simulink model "hyd_hyb_2_int_cont_Final_AMT"  (R2013b)
settings: Solver=ode4  StartTime=0  StopTime=3005  FixedStep=0.01  MaxStep=.4  RelTol=1e-8
InitFcn:
  | const_3_new
values from neighbouring files (symbols this model uses):
  Af = 6.3    [brk_enrg.m]    (also in brk_enrg_1.m)
  BSFC_906_205 = [3.5684 4.3466 5.1668 6.0769 6.988 7.8992 8.8104 9.7336 10.8548 11.9809 13.1112 14.2571 ... (663 elements, 39x17)]    [BSFC_map_906_205.mat]
  Cd = 0.55    [brk_enrg.m]    (also in brk_enrg_1.m)
  den = 1.202    [brk_enrg.m]    (also in brk_enrg_1.m)
  fr = 0.01    [brk_enrg.m]    (also in brk_enrg_1.m)
undefined symbols (not defined in the file or in its folder): clutchRise, down_spd_2, down_spd_3, down_spd_4, down_spd_c, Driving_Cycle, fuel_density, gearshift, I_wheel, Idle_spd_eng_906, M1_hydr, p_v_15, pmax_125, qv_125, Rw, sec_eng_sfc_map, T0, T1, T_max_906, T_min, TC_spd_ratio_max, teta_new_10, torque_convertor, Twait, up_spd_1, up_spd_2, up_spd_3, up_spd_c, v_p_10, v_p_15, v_p_5
libraries: neural x1742, fl_lib x43, nesl_utility x30, sdl_lib x14, simulink x4, simulink_need_slupdate x1
(part 3 of 26)

== system hyd_hyb_2_int_cont_Final_AMT/Transmission1/gear box/gear box/Clutch Control ==
  control : Inport
  1 : Constant
  2 : Constant  Value=2
  3 : Constant  Value=3
  4 : Constant  Value=4
  Add{,1..3} (4 alike) : Sum  Inputs=+-
  Enabled Subsystem1 : Subsystem  TreatAsAtomicUnit=on
  Enabled Subsystem2 : Subsystem  TreatAsAtomicUnit=on
  Enabled Subsystem3 : Subsystem  TreatAsAtomicUnit=on
  Enabled Subsystem4 : Subsystem  TreatAsAtomicUnit=on
  Mux2 : Mux
  disengahe : Constant  Value=-1
  engage : Constant
  selector{1..4} (4 alike) : Switch  Criteria=u2 ~= 0  Threshold=2300  ZeroCross=off
  Clutches : Outport
  wires:
  Mux2/1 -> Clutches/1
  engage/1 -> [engage]
  [disengage] -> selector1/1
  disengahe/1 -> [disengage]
  [engage] -> selector1/3
  control/1 -> Add/1, Add1/1, Add2/1, Add3/1
  Add/1 -> selector1/2
  1/1 -> Add/2
  [disengage] -> selector2/1
  [engage] -> selector2/3
  Add1/1 -> selector2/2
  2/1 -> Add1/2
  [disengage] -> selector3/1
  [engage] -> selector3/3
  Add2/1 -> selector3/2
  3/1 -> Add2/2
  [disengage] -> selector4/1
  [engage] -> selector4/3
  Add3/1 -> selector4/2
  4/1 -> Add3/2
  selector1/1 -> Enabled Subsystem1/Enable
  selector2/1 -> Enabled Subsystem2/Enable
  selector3/1 -> Enabled Subsystem3/Enable
  selector4/1 -> Enabled Subsystem4/Enable
  Enabled Subsystem1/1(clutch release) -> Mux2/1
  Enabled Subsystem2/1(clutch release) -> Mux2/2
  Enabled Subsystem3/1(clutch release) -> Mux2/3
  Enabled Subsystem4/1(clutch release) -> Mux2/4

== system hyd_hyb_2_int_cont_Final_AMT/controller1/online_fuz_clust/online_fuz_clus_main/new_feature_gen1 ==
  mem : Inport
  Clock : Clock
  MATLAB Function : MATLAB Function  TreatAsAtomicUnit=on
  Memory : Memory
  prc_spd_0_10 : Outport
  prc_spd_20_30 : Outport  Port=2
  max_acc : Outport  Port=3
  prc_acc_02_04 : Outport  Port=4
  prc_acc_06_08 : Outport  Port=5
  prc_dec_02_04 : Outport  Port=6
  prc_dec_06_08 : Outport  Port=7
  RPA : Outport  Port=8
  prc_spdacc_0_5 : Outport  Port=9
  PKE : Outport  Port=10
  wires:
  Clock/1 -> MATLAB Function/1(t)
  MATLAB Function/1(prc_spd_0_10) -> prc_spd_0_10/1
  MATLAB Function/2(prc_spd_20_30) -> prc_spd_20_30/1
  MATLAB Function/3(max_acc) -> max_acc/1
  MATLAB Function/4(prc_acc_02_04) -> prc_acc_02_04/1
  MATLAB Function/5(prc_acc_06_08) -> prc_acc_06_08/1
  MATLAB Function/6(prc_dec_02_04) -> prc_dec_02_04/1
  MATLAB Function/7(prc_dec_06_08) -> prc_dec_06_08/1
  MATLAB Function/8(rpa) -> RPA/1
  MATLAB Function/9(prc_av_0_5) -> prc_spdacc_0_5/1
  MATLAB Function/10(pke) -> PKE/1
  Memory/1 -> MATLAB Function/2(mem)
  mem/1 -> Memory/1

== system hyd_hyb_2_int_cont_Final_AMT/controller1/optimized controller/SOC under 0.5/col_c_d ==
  inps : Inport
  SOC : Inport  Port=2
  Switch : Switch  Criteria=u2 > Threshold  Threshold=0.4
  net_col_c_d_2_4 : Subsystem
  net_col_c_d_4_5 : Subsystem
  Out1 : Outport
  wires:
  inps/1 -> net_col_c_d_4_5/1(Input), net_col_c_d_2_4/1(Input)
  SOC/1 -> Switch/2
  net_col_c_d_4_5/1(Output) -> Switch/1
  net_col_c_d_2_4/1(Output) -> Switch/3
  Switch/1 -> Out1/1

== system hyd_hyb_2_int_cont_Final_AMT/controller1/optimized controller/SOC under 0.5/col_c_d1 ==
  inps : Inport
  SOC : Inport  Port=2
  Switch : Switch  Criteria=u2 > Threshold  Threshold=0.4
  net_col_c_d_2_4 : Subsystem
  net_col_c_d_4_5 : Subsystem
  Out1 : Outport
  wires:
  Switch/1 -> Out1/1
  net_col_c_d_2_4/1(Output) -> Switch/3
  net_col_c_d_4_5/1(Output) -> Switch/1
  SOC/1 -> Switch/2
  inps/1 -> net_col_c_d_2_4/1(Input), net_col_c_d_4_5/1(Input)

== system hyd_hyb_2_int_cont_Final_AMT/controller1/optimized controller/SOC under 0.5/col_e_f ==
  inps : Inport
  SOC : Inport  Port=2
  Switch : Switch  Criteria=u2 > Threshold  Threshold=0.4
  net_col_e_f_2_4 : Subsystem
  net_col_e_f_4_5 : Subsystem
  Out1 : Outport
  wires:
  inps/1 -> net_col_e_f_4_5/1(Input), net_col_e_f_2_4/1(Input)
  SOC/1 -> Switch/2
  net_col_e_f_4_5/1(Output) -> Switch/1
  net_col_e_f_2_4/1(Output) -> Switch/3
  Switch/1 -> Out1/1

== system hyd_hyb_2_int_cont_Final_AMT/controller1/optimized controller/SOC under 0.5/net_loc_rod_2_5 ==
  Input : Inport  PortDimensions=2
  Layer 1 : Subsystem
  Layer 2 : Subsystem
  Layer 3 : Subsystem
  Process Input 1 : Subsystem
  Process Output 1 : Subsystem
  Output : Outport  InitialOutput=0
  wires:
  Input/1 -> Process Input 1/1(x)
  Process Output 1/1(y) -> Output/1
  Process Input 1/1(p) -> Layer 1/1("p{1}")
  Layer 1/1("a{1}") -> [feedback1]
  [feedback1] -> Layer 2/1("a{1} ")
  Layer 2/1("a{2}") -> [feedback2]
  [feedback2] -> Layer 3/1("a{2} ")
  Layer 3/1("a{3}") -> Process Output 1/1(a)

== system hyd_hyb_2_int_cont_Final_AMT/controller1/optimized controller/SOC upper 0.5/SOC under 0.6 ==
  inps : Inport
  u_fuzz : Inport  Port=2
  Action Port : ActionPort  ActionType=then
  Demux : Demux
  Product{,1..3} (4 alike) : Product  RndMeth=Zero
  Saturation{1..4} (4 alike) : Saturate  UpperLimit=1  LowerLimit=0
  Sum : Sum  Inputs=++++
  net_col_a_b_5_6 : Subsystem
  net_col_c_d_5_6 : Subsystem
  net_col_e_f_5_6 : Subsystem
  net_loc_rod_5_6 : Subsystem
  T_ICE_opt : Outport
  wires:
  Sum/1 -> T_ICE_opt/1
  inps/1 -> net_col_c_d_5_6/1(Input), net_col_e_f_5_6/1(Input), net_loc_rod_5_6/1(Input), net_col_a_b_5_6/1(Input)
  net_loc_rod_5_6/1(Output) -> Saturation2/1
  Product/1 -> Sum/1
  net_col_c_d_5_6/1(Output) -> Saturation4/1
  net_col_a_b_5_6/1(Output) -> Saturation1/1
  net_col_e_f_5_6/1(Output) -> Saturation3/1
  Saturation2/1 -> Product/1
  Saturation1/1 -> Product1/1
  Saturation4/1 -> Product2/1
  Saturation3/1 -> Product3/1
  Demux/1 -> Product1/2
  Demux/2 -> Product2/2
  u_fuzz/1 -> Demux/1
  Demux/3 -> Product3/2
  Demux/4 -> Product/2
  Product3/1 -> Sum/4
  Product2/1 -> Sum/3
  Product1/1 -> Sum/2

== system hyd_hyb_2_int_cont_Final_AMT/controller1/optimized controller/SOC upper 0.5/SOC upper 0.6 ==
  In1 : Inport
  SOC : Inport  Port=2
  u_fuzz : Inport  Port=3
  Action Port : ActionPort  ActionType=else
  If : If  IfExpression=u1 <=0.7
  SOC under 0.7 : Subsystem  TreatAsAtomicUnit=on
  SOC upper 0.7 : Subsystem  TreatAsAtomicUnit=on
  Switch : Switch  Criteria=u2 > Threshold  Threshold=0.7
  T_ICE_opt : Outport
  wires:
  SOC/1 -> SOC upper 0.7/1(SOC), If/1, Switch/2
  In1/1 -> SOC under 0.7/1(inps), SOC upper 0.7/2(inps)
  If/1 -> SOC under 0.7/Action
  If/2 -> SOC upper 0.7/Action
  Switch/1 -> T_ICE_opt/1
  SOC upper 0.7/1(T_ICE_opt) -> Switch/1
  SOC under 0.7/1(T_ICE_opt) -> Switch/3
  u_fuzz/1 -> SOC under 0.7/2(u_fuzz), SOC upper 0.7/3(u_fuzz)

== system hyd_hyb_2_int_cont_Final_AMT/hydraulic transmission/PM_hydraulic_machine /eta estimator/eta_t ==
  qv : Inport
  delta_p : Inport  Port=2
  Pmax : Inport  Port=3
  Abs : Abs
  Abs1 : Abs
  Constant : Constant  Value=600
  Constant1 : Constant  Value=0
  Divide : Product  Inputs=*/
  Product : Product  RndMeth=Zero
  Product1 : Product  RndMeth=Zero
  Saturation : Saturate  UpperLimit=1  LowerLimit=0
  Saturation1 : Saturate  UpperLimit=inf  LowerLimit=0.0000001
  Scope : Scope
      settings: SaveName=ScopeData29
  Scope1 : Scope  NumInputPorts=2
      settings: TimeRange=2.2  YMin=-5~-5  YMax=5~5  SaveName=ScopeData30
  Scope2 : Scope
      settings: YMin=0  YMax=190  SaveName=ScopeData50
  Scope3 : Scope
      settings: YMin=0  YMax=190  SaveName=ScopeData51
  Switch : Switch  Threshold=1
  eta_t : Outport
  wires:
  qv/1 -> Product1/1, Abs1/1
  delta_p/1 -> Product1/2
  Pmax/1 -> Product/1
  Constant/1 -> Product/2
  Product1/1 -> Abs/1
  Abs/1 -> Divide/1, Scope1/1
  Product/1 -> Saturation1/1
  Abs1/1 -> Scope2/1, Switch/2
  Saturation/1 -> eta_t/1
  Switch/1 -> Saturation/1, Scope/1
  Divide/1 -> Switch/1, Scope3/1
  Constant1/1 -> Switch/3
  Saturation1/1 -> Divide/2, Scope1/2

== system hyd_hyb_2_int_cont_Final_AMT/hydraulic transmission/PM_hydraulic_machine /eta estimator/eta_v ==
  qv : Inport
  vg : Inport  Port=2
  n : Inport  Port=3
  Abs : Abs
  Abs1 : Abs
  Abs2 : Abs
  Constant : Constant  Value=1000
  Constant1 : Constant  Value=0.00001
  Divide : Product  Inputs=*/
  Product : Product  RndMeth=Zero
  Product1 : Product  RndMeth=Zero
  Saturation : Saturate  UpperLimit=1  LowerLimit=0.000001
  Saturation1 : Saturate  UpperLimit=inf  LowerLimit=0.0000001
  Scope : Scope  NumInputPorts=2
      settings: TimeRange=2  YMin=-5~-5  YMax=5~5  SaveName=ScopeData43
  Scope1 : Scope
      settings: TimeRange=2  SaveName=ScopeData44
  Scope2 : Scope  NumInputPorts=2
      settings: TimeRange=2  YMin=-5~-5  YMax=5~5  SaveName=ScopeData45
  Scope3 : Scope  NumInputPorts=2
      settings: TimeRange=2  YMin=-5~-5  YMax=5~5  SaveName=ScopeData46
  Scope4 : Scope
      settings: SaveName=ScopeData52
  Switch : Switch  Threshold=1
  eta_v : Outport
  wires:
  n/1 -> Product/1, Scope2/1
  vg/1 -> Product/2, Scope2/2
  qv/1 -> Scope3/1, Product1/1, Abs2/1
  Constant/1 -> Product1/2
  Product1/1 -> Abs/1
  Abs/1 -> Divide/1, Scope/1
  Product/1 -> Abs1/1
  Abs1/1 -> Scope/2, Saturation1/1
  Divide/1 -> Switch/1, Scope4/1
  Constant1/1 -> Switch/3
  Switch/1 -> Saturation/1, Scope1/1
  Saturation/1 -> eta_v/1
  Abs2/1 -> Switch/2
  Saturation1/1 -> Divide/2

== system hyd_hyb_2_int_cont_Final_AMT/hydraulic transmission/accumulator/max - min volume estimator/for 10 gal accumulator ==
  min_press(psi) : Inport
  max_press(psi) : Inport  Port=2
  pre_ch_press(psi) : Inport  Port=3
  Action Port : ActionPort  PropagateVarSize=During execution  ActionType=then
  Constant : Constant  Value=152
  Scope : Scope  NumInputPorts=2
      settings: YMin=-5~-5  YMax=5~5  SaveName=ScopeData40
  Scope1 : Scope  NumInputPorts=2
      settings: YMin=-5~-5  YMax=5~5  SaveName=ScopeData41
  in^3 to lit : Gain  Gain=16.387e-3
  in^3 to lit (1) : Gain  Gain=16.387e-3
  rexroth-1 : Lookup_n-D  BreakpointsForDimension1=[1000,1100,1200,1300,1400,1500,1600,1700,1800,1900,2000,2100,2200,2300,2400,2500,2600,2700,2800,2900,3000,3100,3200,3300,3400,3500,3600,3700,3800,3900,4000,4100,4200,4300,4400,4500,4600,4700,4800,4900,5000,5100,5200,5300,5400,5500,5600,5700,5800,5900,6000]  BreakpointsForDimension2=[1000,1400,2000]  Table=v_p_10  InputSameDT=on
  rexroth-10 : Lookup_n-D  BreakpointsForDimension1=[1000,1100,1200,1300,1400,1500,1600,1700,1800,1900,2000,2100,2200,2300,2400,2500,2600,2700,2800,2900,3000,3100,3200,3300,3400,3500,3600,3700,3800,3900,4000,4100,4200,4300,4400,4500,4600,4700,4800,4900,5000,5100,5200,5300,5400,5500,5600,5700,5800,5900,6000]  BreakpointsForDimension2=[1000,1400,2000]  Table=v_p_10  InputSameDT=on
  min_vol(lit) : Outport
  max_vol(lit) : Outport  Port=2
  accum_dry_mass ( kg ) : Outport  Port=3  InitialOutput=[0]
  wires:
  in^3 to lit/1 -> min_vol(lit)/1, Scope1/1
  rexroth-10/1 -> in^3 to lit (1)/1, Scope/2
  rexroth-1/1 -> in^3 to lit/1, Scope/1
  in^3 to lit (1)/1 -> max_vol(lit)/1, Scope1/2
  pre_ch_press(psi)/1 -> rexroth-10/2, rexroth-1/2
  min_press(psi)/1 -> rexroth-1/1
  max_press(psi)/1 -> rexroth-10/1
  Constant/1 -> accum_dry_mass ( kg )/1

== system hyd_hyb_2_int_cont_Final_AMT/hydraulic transmission/accumulator/max - min volume estimator/for 15 gal accumulator1 ==
  min_press(psi) : Inport
  max_press(psi) : Inport  Port=2
  pre_ch_press(psi) : Inport  Port=3
  Action Port : ActionPort  PropagateVarSize=During execution  ActionType=then
  Constant : Constant  Value=220
  Scope : Scope  NumInputPorts=2
      settings: YMin=-5~-5  YMax=5~5  SaveName=ScopeData38
  Scope1 : Scope  NumInputPorts=2
      settings: YMin=4.74484~24.0403  YMax=4.74484~24.0403  SaveName=ScopeData39
  in^3 to lit : Gain  Gain=16.387e-3
  in^3 to lit (1) : Gain  Gain=16.387e-3
  rexroth-1 : Lookup_n-D  BreakpointsForDimension1=[1000,1100,1200,1300,1400,1500,1600,1700,1800,1900,2000,2100,2200,2300,2400,2500,2600,2700,2800,2900,3000,3100,3200,3300,3400,3500,3600,3700,3800,3900,4000,4100,4200,4300,4400,4500,4600,4700,4800,4900,5000,5100,5200,5300,5400,5500,5600,5700,5800,5900,6000]  BreakpointsForDimension2=[1000,1400,2000]  Table=v_p_15  InputSameDT=on
  rexroth-15 : Lookup_n-D  BreakpointsForDimension1=[1000,1100,1200,1300,1400,1500,1600,1700,1800,1900,2000,2100,2200,2300,2400,2500,2600,2700,2800,2900,3000,3100,3200,3300,3400,3500,3600,3700,3800,3900,4000,4100,4200,4300,4400,4500,4600,4700,4800,4900,5000,5100,5200,5300,5400,5500,5600,5700,5800,5900,6000]  BreakpointsForDimension2=[1000,1400,2000]  Table=v_p_15  InputSameDT=on
  min_vol(lit) : Outport
  max_vol(lit) : Outport  Port=2
  accum_dry_mass ( kg ) : Outport  Port=3  InitialOutput=[0]
  wires:
  in^3 to lit/1 -> min_vol(lit)/1, Scope1/1
  rexroth-1/1 -> in^3 to lit (1)/1, Scope/2
  rexroth-15/1 -> in^3 to lit/1, Scope/1
  in^3 to lit (1)/1 -> max_vol(lit)/1, Scope1/2
  pre_ch_press(psi)/1 -> rexroth-15/2, rexroth-1/2
  min_press(psi)/1 -> rexroth-15/1
  max_press(psi)/1 -> rexroth-1/1
  Constant/1 -> accum_dry_mass ( kg )/1

== system hyd_hyb_2_int_cont_Final_AMT/hydraulic transmission/accumulator/max - min volume estimator/for 5 gal accumulator ==
  min_press(psi) : Inport
  max_press(psi) : Inport  Port=2
  pre_ch_press(psi) : Inport  Port=3
  Action Port : ActionPort  PropagateVarSize=During execution  ActionType=then
  Constant : Constant  Value=100
  Scope : Scope  NumInputPorts=2
      settings: YMin=-5~-5  YMax=5~5  SaveName=ScopeData27
  Scope1 : Scope  NumInputPorts=2
      settings: YMin=61.8714~626.852  YMax=61.8714~626.852  SaveName=ScopeData28
  in^3 to lit : Gain  Gain=16.387e-3
  in^3 to lit (1) : Gain  Gain=16.387e-3
  rexroth-1 : Lookup_n-D  BreakpointsForDimension1=[1000,1100,1200,1300,1400,1500,1600,1700,1800,1900,2000,2100,2200,2300,2400,2500,2600,2700,2800,2900,3000,3100,3200,3300,3400,3500,3600,3700,3800,3900,4000,4100,4200,4300,4400,4500,4600,4700,4800,4900,5000,5100,5200,5300,5400,5500,5600,5700,5800,5900,6000]  BreakpointsForDimension2=[1000,1400,2000]  Table=v_p_5  InputSameDT=on
  rexroth-5 : Lookup_n-D  BreakpointsForDimension1=[1000,1100,1200,1300,1400,1500,1600,1700,1800,1900,2000,2100,2200,2300,2400,2500,2600,2700,2800,2900,3000,3100,3200,3300,3400,3500,3600,3700,3800,3900,4000,4100,4200,4300,4400,4500,4600,4700,4800,4900,5000,5100,5200,5300,5400,5500,5600,5700,5800,5900,6000]  BreakpointsForDimension2=[1000,1400,2000]  Table=v_p_5  InputSameDT=on
  min_vol(lit) : Outport
  max_vol(lit) : Outport  Port=2
  accum_dry_mass ( kg ) : Outport  Port=3  InitialOutput=[0]
  wires:
  in^3 to lit/1 -> min_vol(lit)/1, Scope/1
  rexroth-1/1 -> in^3 to lit (1)/1, Scope1/2
  rexroth-5/1 -> in^3 to lit/1, Scope1/1
  in^3 to lit (1)/1 -> max_vol(lit)/1, Scope/2
  pre_ch_press(psi)/1 -> rexroth-5/2, rexroth-1/2
  min_press(psi)/1 -> rexroth-5/1
  max_press(psi)/1 -> rexroth-1/1
  Constant/1 -> accum_dry_mass ( kg )/1

== system hyd_hyb_2_int_cont_Final_AMT/Transmission1/Torque Convertor/main solver/Sensor(TC_in)/Motion sensor ==
  Ideal Rotational Motion Sensor : fl_lib/Mechanical/Mechanical Sensors/Ideal Rotational Motion Sensor  offset=0 rad  w_Log=off  t_Log=off  phi_Log=off  LocalVarNames=|w|t|phi  LocalVarDescs=|w|t|phi  LocalVarLogging=[]
  MRR : fl_lib/Mechanical/Rotational Elements/Mechanical Rotational Reference  t_Log=off  LocalVarNames=|t  LocalVarDescs=|t  LocalVarLogging=[]
  PS-Simulink Converter : nesl_utility/PS-Simulink Converter  PhysicalDomain=network_engine_domain  SubClassName=ps_output  LeftPortType=input  RightPortType=output  PseudoPeriodic=off  Frequencies=[]  Unit=rad/s  AffineConversion=off
  A : PMIOPort  Port=1  Side=Left
  W : Outport
  wires:
  PS-Simulink Converter/1 -> W/1
  connections:
  A/RConn1 -- Ideal Rotational Motion Sensor/LConn1
  Ideal Rotational Motion Sensor/RConn2 -- PS-Simulink Converter/LConn1
  MRR/LConn1 -- Ideal Rotational Motion Sensor/RConn1

== system hyd_hyb_2_int_cont_Final_AMT/Transmission1/Torque Convertor/main solver/Sensor(TC_in)/Torque sensor ==
  PS2S : nesl_utility/PS-Simulink Converter  PhysicalDomain=network_engine_domain  SubClassName=ps_output  LeftPortType=input  RightPortType=output  PseudoPeriodic=off  Frequencies=[]  Unit=1  AffineConversion=off
  Torque Sensor : fl_lib/Mechanical/Mechanical Sensors/Ideal Torque Sensor  w_Log=off  t_Log=off  LocalVarNames=|w|t  LocalVarDescs=|w|t  LocalVarLogging=[]
  B : PMIOPort  Port=1  Side=Right
  A : PMIOPort  Port=2  Side=Left
  T : Outport
  wires:
  PS2S/1 -> T/1
  connections:
  A/RConn1 -- Torque Sensor/LConn1
  B/RConn1 -- Torque Sensor/RConn1
  Torque Sensor/RConn2 -- PS2S/LConn1

== system hyd_hyb_2_int_cont_Final_AMT/Transmission1/Torque Convertor/main solver/Sensor(TC_out)/Motion sensor ==
  Ideal Rotational Motion Sensor : fl_lib/Mechanical/Mechanical Sensors/Ideal Rotational Motion Sensor  offset=0 rad  w_Log=off  t_Log=off  phi_Log=off  LocalVarNames=|w|t|phi  LocalVarDescs=|w|t|phi  LocalVarLogging=[]
  MRR : fl_lib/Mechanical/Rotational Elements/Mechanical Rotational Reference  t_Log=off  LocalVarNames=|t  LocalVarDescs=|t  LocalVarLogging=[]
  PS-Simulink Converter : nesl_utility/PS-Simulink Converter  PhysicalDomain=network_engine_domain  SubClassName=ps_output  LeftPortType=input  RightPortType=output  PseudoPeriodic=off  Frequencies=[]  Unit=rad/s  AffineConversion=off
  A : PMIOPort  Port=1  Side=Left
  W : Outport
  wires:
  PS-Simulink Converter/1 -> W/1
  connections:
  MRR/LConn1 -- Ideal Rotational Motion Sensor/RConn1
  Ideal Rotational Motion Sensor/RConn2 -- PS-Simulink Converter/LConn1
  A/RConn1 -- Ideal Rotational Motion Sensor/LConn1

== system hyd_hyb_2_int_cont_Final_AMT/Transmission1/Torque Convertor/main solver/Sensor(TC_out)/Torque sensor ==
  PS2S : nesl_utility/PS-Simulink Converter  PhysicalDomain=network_engine_domain  SubClassName=ps_output  LeftPortType=input  RightPortType=output  PseudoPeriodic=off  Frequencies=[]  Unit=1  AffineConversion=off
  Torque Sensor : fl_lib/Mechanical/Mechanical Sensors/Ideal Torque Sensor  w_Log=off  t_Log=off  LocalVarNames=|w|t  LocalVarDescs=|w|t  LocalVarLogging=[]
  B : PMIOPort  Port=1  Side=Right
  A : PMIOPort  Port=2  Side=Left
  T : Outport
  wires:
  PS2S/1 -> T/1
  connections:
  Torque Sensor/RConn2 -- PS2S/LConn1
  B/RConn1 -- Torque Sensor/RConn1
  A/RConn1 -- Torque Sensor/LConn1

== system hyd_hyb_2_int_cont_Final_AMT/Transmission1/gear box/gear box/Clutch Control/Enabled Subsystem1 ==
  Enable : EnablePort  StatesWhenEnabling=reset  PropagateVarSize=During execution
  Clutch A Actuator : TransferFcn  Numerator=[1/clutchRise]  Denominator=[1 1/clutchRise]
  engage : Constant
  clutch release : Outport  OutputWhenDisabled=reset  InitialOutput=[0]
  wires:
  engage/1 -> Clutch A Actuator/1
  Clutch A Actuator/1 -> clutch release/1

== system hyd_hyb_2_int_cont_Final_AMT/Transmission1/gear box/gear box/Clutch Control/Enabled Subsystem2 ==
  Enable : EnablePort  StatesWhenEnabling=reset  PropagateVarSize=During execution
  Clutch A Actuator : TransferFcn  Numerator=[1/clutchRise]  Denominator=[1 1/clutchRise]
  engage : Constant
  clutch release : Outport  OutputWhenDisabled=reset  InitialOutput=[0]
  wires:
  Clutch A Actuator/1 -> clutch release/1
  engage/1 -> Clutch A Actuator/1

== system hyd_hyb_2_int_cont_Final_AMT/Transmission1/gear box/gear box/Clutch Control/Enabled Subsystem3 ==
  Enable : EnablePort  StatesWhenEnabling=reset  PropagateVarSize=During execution
  Clutch A Actuator : TransferFcn  Numerator=[1/clutchRise]  Denominator=[1 1/clutchRise]
  engage : Constant
  clutch release : Outport  OutputWhenDisabled=reset  InitialOutput=[0]
  wires:
  engage/1 -> Clutch A Actuator/1
  Clutch A Actuator/1 -> clutch release/1

== system hyd_hyb_2_int_cont_Final_AMT/Transmission1/gear box/gear box/Clutch Control/Enabled Subsystem4 ==
  Enable : EnablePort  StatesWhenEnabling=reset  PropagateVarSize=During execution
  Clutch A Actuator : TransferFcn  Numerator=[1/clutchRise]  Denominator=[1 1/clutchRise]
  engage : Constant
  clutch release : Outport  OutputWhenDisabled=reset  InitialOutput=[0]
  wires:
  Clutch A Actuator/1 -> clutch release/1
  engage/1 -> Clutch A Actuator/1

== system hyd_hyb_2_int_cont_Final_AMT/controller1/optimized controller/SOC under 0.5/col_c_d/net_col_c_d_2_4 ==
  Input : Inport  PortDimensions=2
  Layer 1 : Subsystem
  Layer 2 : Subsystem
  Layer 3 : Subsystem
  Process Input 1 : Subsystem
  Process Output 1 : Subsystem
  Output : Outport  InitialOutput=0
  wires:
  Input/1 -> Process Input 1/1(x)
  Process Output 1/1(y) -> Output/1
  Process Input 1/1(p) -> Layer 1/1("p{1}")
  Layer 1/1("a{1}") -> [feedback1]
  [feedback1] -> Layer 2/1("a{1} ")
  Layer 2/1("a{2}") -> [feedback2]
  [feedback2] -> Layer 3/1("a{2} ")
  Layer 3/1("a{3}") -> Process Output 1/1(a)

== system hyd_hyb_2_int_cont_Final_AMT/controller1/optimized controller/SOC under 0.5/col_c_d/net_col_c_d_4_5 ==
  Input : Inport  PortDimensions=2
  Layer 1 : Subsystem
  Layer 2 : Subsystem
  Layer 3 : Subsystem
  Process Input 1 : Subsystem
  Process Output 1 : Subsystem
  Output : Outport  InitialOutput=0
  wires:
  Input/1 -> Process Input 1/1(x)
  Process Output 1/1(y) -> Output/1
  Process Input 1/1(p) -> Layer 1/1("p{1}")
  Layer 1/1("a{1}") -> [feedback1]
  [feedback1] -> Layer 2/1("a{1} ")
  Layer 2/1("a{2}") -> [feedback2]
  [feedback2] -> Layer 3/1("a{2} ")
  Layer 3/1("a{3}") -> Process Output 1/1(a)

== system hyd_hyb_2_int_cont_Final_AMT/controller1/optimized controller/SOC under 0.5/col_c_d1/net_col_c_d_2_4 ==
  Input : Inport  PortDimensions=2
  Layer 1 : Subsystem
  Layer 2 : Subsystem
  Layer 3 : Subsystem
  Process Input 1 : Subsystem
  Process Output 1 : Subsystem
  Output : Outport  InitialOutput=0
  wires:
  Layer 3/1("a{3}") -> Process Output 1/1(a)
  [feedback2] -> Layer 3/1("a{2} ")
  Layer 2/1("a{2}") -> [feedback2]
  [feedback1] -> Layer 2/1("a{1} ")
  Layer 1/1("a{1}") -> [feedback1]
  Process Input 1/1(p) -> Layer 1/1("p{1}")
  Process Output 1/1(y) -> Output/1
  Input/1 -> Process Input 1/1(x)

== system hyd_hyb_2_int_cont_Final_AMT/controller1/optimized controller/SOC under 0.5/col_c_d1/net_col_c_d_4_5 ==
  Input : Inport  PortDimensions=2
  Layer 1 : Subsystem
  Layer 2 : Subsystem
  Layer 3 : Subsystem
  Process Input 1 : Subsystem
  Process Output 1 : Subsystem
  Output : Outport  InitialOutput=0
  wires:
  Layer 3/1("a{3}") -> Process Output 1/1(a)
  [feedback2] -> Layer 3/1("a{2} ")
  Layer 2/1("a{2}") -> [feedback2]
  [feedback1] -> Layer 2/1("a{1} ")
  Layer 1/1("a{1}") -> [feedback1]
  Process Input 1/1(p) -> Layer 1/1("p{1}")
  Process Output 1/1(y) -> Output/1
  Input/1 -> Process Input 1/1(x)

== system hyd_hyb_2_int_cont_Final_AMT/controller1/optimized controller/SOC under 0.5/col_e_f/net_col_e_f_2_4 ==
  Input : Inport  PortDimensions=2
  Layer 1 : Subsystem
  Layer 2 : Subsystem
  Layer 3 : Subsystem
  Process Input 1 : Subsystem
  Process Output 1 : Subsystem
  Output : Outport  InitialOutput=0
  wires:
  Input/1 -> Process Input 1/1(x)
  Process Output 1/1(y) -> Output/1
  Process Input 1/1(p) -> Layer 1/1("p{1}")
  Layer 1/1("a{1}") -> [feedback1]
  [feedback1] -> Layer 2/1("a{1} ")
  Layer 2/1("a{2}") -> [feedback2]
  [feedback2] -> Layer 3/1("a{2} ")
  Layer 3/1("a{3}") -> Process Output 1/1(a)

== system hyd_hyb_2_int_cont_Final_AMT/controller1/optimized controller/SOC under 0.5/col_e_f/net_col_e_f_4_5 ==
  Input : Inport  PortDimensions=2
  Layer 1 : Subsystem
  Layer 2 : Subsystem
  Layer 3 : Subsystem
  Process Input 1 : Subsystem
  Process Output 1 : Subsystem
  Output : Outport  InitialOutput=0
  wires:
  Input/1 -> Process Input 1/1(x)
  Process Output 1/1(y) -> Output/1
  Process Input 1/1(p) -> Layer 1/1("p{1}")
  Layer 1/1("a{1}") -> [feedback1]
  [feedback1] -> Layer 2/1("a{1} ")
  Layer 2/1("a{2}") -> [feedback2]
  [feedback2] -> Layer 3/1("a{2} ")
  Layer 3/1("a{3}") -> Process Output 1/1(a)

== system hyd_hyb_2_int_cont_Final_AMT/controller1/optimized controller/SOC under 0.5/net_loc_rod_2_5/Layer 1 ==
  "p{1}" : Inport  PortDimensions=2
  Delays 1 : Subsystem
  "IW{1,1}" : Subsystem
  "b{1}" : Constant  Value=[-4.427231660818169;3.456636280494104;2.4300449872666854;1.4410928325775507;-0.49232939607411785;-0.49242330153496311;1.5258039114342512;-2.4759475246010565;3.4877744812530702;-4.4171792578500666]
  netsum : Sum  Inputs=2  SaturateOnIntegerOverflow=on  InputSameDT=on  OutDataTypeStr=Inherit: Same as first input
  tansig : neural/Transfer Functions/tansig
  "a{1}" : Outport  InitialOutput=[0;0;0;0;0;0;0;0;0;0]
  wires:
  "p{1}"/1 -> Delays 1/1("p{1}")
  Delays 1/1("pd{1,1}") -> "IW{1,1}"/1("pd{1,1}")
  "IW{1,1}"/1("iz{1,1}") -> netsum/1
  "b{1}"/1 -> netsum/2
  netsum/1 -> tansig/1
  tansig/1 -> "a{1}"/1

== system hyd_hyb_2_int_cont_Final_AMT/controller1/optimized controller/SOC under 0.5/net_loc_rod_2_5/Layer 2 ==
  "a{1} " : Inport  PortDimensions=10
  Delays 1 : Subsystem
  "LW{2,1}" : Subsystem
  "b{2}" : Constant  Value=[-1.8283395045760578;-1.5112791815228035;-1.3096453352155384;0.99927747204973882;-0.87070649425908642;0.57038205764658179;0.26248556891103664;0.037384065008415478;-0.25474765773298769;-0.5223912617711548;0.79462611488080304;0.93340606123125525;-1.2890933117577059;1.5735286477660981;-1.8440196925158161]
  netsum : Sum  Inputs=2  SaturateOnIntegerOverflow=on  InputSameDT=on  OutDataTypeStr=Inherit: Same as first input
  tansig : neural/Transfer Functions/tansig
  "a{2}" : Outport  InitialOutput=[0;0;0;0;0;0;0;0;0;0;0;0;0;0;0]
  wires:
  "a{1} "/1 -> Delays 1/1("p{2}")
  Delays 1/1("pd{2,1}") -> "LW{2,1}"/1("ad{2,1}")
  "LW{2,1}"/1("lz{2,1}") -> netsum/1
  "b{2}"/1 -> netsum/2
  netsum/1 -> tansig/1
  tansig/1 -> "a{2}"/1

== system hyd_hyb_2_int_cont_Final_AMT/controller1/optimized controller/SOC under 0.5/net_loc_rod_2_5/Layer 3 ==
  "a{2} " : Inport  PortDimensions=15
  Delays 1 : Subsystem
  "LW{3,2}" : Subsystem
  "b{3}" : Constant  Value=0.060410481787306604
  netsum : Sum  Inputs=2  SaturateOnIntegerOverflow=on  InputSameDT=on  OutDataTypeStr=Inherit: Same as first input
  purelin : neural/Transfer Functions/purelin
  "a{3}" : Outport  InitialOutput=0
  wires:
  "a{2} "/1 -> Delays 1/1("p{3}")
  Delays 1/1("pd{3,2}") -> "LW{3,2}"/1("ad{3,2}")
  "LW{3,2}"/1("lz{3,2}") -> netsum/1
  "b{3}"/1 -> netsum/2
  netsum/1 -> purelin/1
  purelin/1 -> "a{3}"/1

== system hyd_hyb_2_int_cont_Final_AMT/controller1/optimized controller/SOC under 0.5/net_loc_rod_2_5/Process Input 1 ==
  x : Inport  PortDimensions=2
  fixunknowns : neural/Processing Functions/fixunknowns  inputSize=2  indices=[1 2]
  mapminmax : neural/Processing Functions/mapminmax  xmin=[0.0022593599778436804;0.375]  xmax=[1;0.48752699999999999]  ymin=-1  ymax=1
  removeconstantrows : neural/Processing Functions/removeconstantrows  inputSize=2  keep=[1 2]
  p : Outport  PortDimensions=2
  wires:
  x/1 -> fixunknowns/1
  fixunknowns/1 -> removeconstantrows/1
  removeconstantrows/1 -> mapminmax/1
  mapminmax/1 -> p/1

== system hyd_hyb_2_int_cont_Final_AMT/controller1/optimized controller/SOC under 0.5/net_loc_rod_2_5/Process Output 1 ==
  a : Inport  PortDimensions=1
  mapminmax_reverse : neural/Processing Functions/mapminmax_reverse  xmin=0  xmax=0.71867283838575113  ymin=-1  ymax=1
  removeconstantrows_reverse : neural/Processing Functions/removeconstantrows_reverse  inputSize=1  constants=zeros(0,1)  rearrange=1
  y : Outport  PortDimensions=1
  wires:
  a/1 -> mapminmax_reverse/1
  mapminmax_reverse/1 -> removeconstantrows_reverse/1
  removeconstantrows_reverse/1 -> y/1

== system hyd_hyb_2_int_cont_Final_AMT/controller1/optimized controller/SOC upper 0.5/SOC under 0.6/net_col_a_b_5_6 ==
  Input : Inport  PortDimensions=2
  Layer 1 : Subsystem
  Layer 2 : Subsystem
  Layer 3 : Subsystem
  Process Input 1 : Subsystem
  Process Output 1 : Subsystem
  Output : Outport  InitialOutput=0
  wires:
  Input/1 -> Process Input 1/1(x)
  Process Output 1/1(y) -> Output/1
  Process Input 1/1(p) -> Layer 1/1("p{1}")
  Layer 1/1("a{1}") -> [feedback1]
  [feedback1] -> Layer 2/1("a{1} ")
  Layer 2/1("a{2}") -> [feedback2]
  [feedback2] -> Layer 3/1("a{2} ")
  Layer 3/1("a{3}") -> Process Output 1/1(a)

== system hyd_hyb_2_int_cont_Final_AMT/controller1/optimized controller/SOC upper 0.5/SOC under 0.6/net_col_c_d_5_6 ==
  Input : Inport  PortDimensions=2
  Layer 1 : Subsystem
  Layer 2 : Subsystem
  Layer 3 : Subsystem
  Process Input 1 : Subsystem
  Process Output 1 : Subsystem
  Output : Outport  InitialOutput=0
  wires:
  Input/1 -> Process Input 1/1(x)
  Process Output 1/1(y) -> Output/1
  Process Input 1/1(p) -> Layer 1/1("p{1}")
  Layer 1/1("a{1}") -> [feedback1]
  [feedback1] -> Layer 2/1("a{1} ")
  Layer 2/1("a{2}") -> [feedback2]
  [feedback2] -> Layer 3/1("a{2} ")
  Layer 3/1("a{3}") -> Process Output 1/1(a)

== system hyd_hyb_2_int_cont_Final_AMT/controller1/optimized controller/SOC upper 0.5/SOC under 0.6/net_col_e_f_5_6 ==
  Input : Inport  PortDimensions=2
  Layer 1 : Subsystem
  Layer 2 : Subsystem
  Layer 3 : Subsystem
  Process Input 1 : Subsystem
  Process Output 1 : Subsystem
  Output : Outport  InitialOutput=0
  wires:
  Input/1 -> Process Input 1/1(x)
  Process Output 1/1(y) -> Output/1
  Process Input 1/1(p) -> Layer 1/1("p{1}")
  Layer 1/1("a{1}") -> [feedback1]
  [feedback1] -> Layer 2/1("a{1} ")
  Layer 2/1("a{2}") -> [feedback2]
  [feedback2] -> Layer 3/1("a{2} ")
  Layer 3/1("a{3}") -> Process Output 1/1(a)

== system hyd_hyb_2_int_cont_Final_AMT/controller1/optimized controller/SOC upper 0.5/SOC under 0.6/net_loc_rod_5_6 ==
  Input : Inport  PortDimensions=2
  Layer 1 : Subsystem
  Layer 2 : Subsystem
  Layer 3 : Subsystem
  Process Input 1 : Subsystem
  Process Output 1 : Subsystem
  Output : Outport  InitialOutput=0
  wires:
  Input/1 -> Process Input 1/1(x)
  Process Output 1/1(y) -> Output/1
  Process Input 1/1(p) -> Layer 1/1("p{1}")
  Layer 1/1("a{1}") -> [feedback1]
  [feedback1] -> Layer 2/1("a{1} ")
  Layer 2/1("a{2}") -> [feedback2]
  [feedback2] -> Layer 3/1("a{2} ")
  Layer 3/1("a{3}") -> Process Output 1/1(a)

== system hyd_hyb_2_int_cont_Final_AMT/controller1/optimized controller/SOC upper 0.5/SOC upper 0.6/SOC under 0.7 ==
  inps : Inport
  u_fuzz : Inport  Port=2
  Action Port : ActionPort  ActionType=then
  Demux : Demux
  Product{,1..3} (4 alike) : Product  RndMeth=Zero
  Saturation{1..4} (4 alike) : Saturate  UpperLimit=1  LowerLimit=0
  Sum : Sum  Inputs=++++
  net_col_a_b_6_1 : Subsystem
  net_col_a_b_6_7 : Subsystem
  net_col_e_f_6_7 : Subsystem
  net_loc_rod_6_7 : Subsystem
  T_ICE_opt : Outport
  wires:
  Sum/1 -> T_ICE_opt/1
  inps/1 -> net_loc_rod_6_7/1(Input), net_col_a_b_6_7/1(Input), net_col_a_b_6_1/1(Input), net_col_e_f_6_7/1(Input)
  net_loc_rod_6_7/1(Output) -> Saturation2/1
  Product/1 -> Sum/1
  Product1/1 -> Sum/2
  Product2/1 -> Sum/3
  Product3/1 -> Sum/4
  net_col_a_b_6_1/1(Output) -> Saturation3/1
  net_col_a_b_6_7/1(Output) -> Saturation1/1
  net_col_e_f_6_7/1(Output) -> Saturation4/1
  Saturation2/1 -> Product/1
  Saturation1/1 -> Product1/1
  Saturation3/1 -> Product2/1
  Saturation4/1 -> Product3/1
  Demux/1 -> Product1/2
  Demux/2 -> Product2/2
  Demux/3 -> Product3/2
  Demux/4 -> Product/2
  u_fuzz/1 -> Demux/1

== system hyd_hyb_2_int_cont_Final_AMT/controller1/optimized controller/SOC upper 0.5/SOC upper 0.6/SOC upper 0.7 ==
  SOC : Inport
  inps : Inport  Port=2
  u_fuzz : Inport  Port=3
  Action Port : ActionPort  ActionType=else
  If : If  IfExpression=u1 <=0.8
  SOC under 0.8 : Subsystem  TreatAsAtomicUnit=on
  SOC upper 0.8 : Subsystem  TreatAsAtomicUnit=on
  Switch : Switch  Criteria=u2 > Threshold  Threshold=0.8
  T_ICE_opt : Outport
  wires:
  SOC/1 -> If/1, Switch/2
  If/1 -> SOC under 0.8/Action
  If/2 -> SOC upper 0.8/Action
  inps/1 -> SOC under 0.8/1(inps), SOC upper 0.8/1(inps)
  SOC under 0.8/1(T_ICE_opt) -> Switch/3
  SOC upper 0.8/1(T_ICE_opt) -> Switch/1
  Switch/1 -> T_ICE_opt/1
  u_fuzz/1 -> SOC under 0.8/2(u_fuzz), SOC upper 0.8/2(u_fuzz)

== system hyd_hyb_2_int_cont_Final_AMT/controller1/optimized controller/SOC under 0.5/col_c_d/net_col_c_d_2_4/Layer 1 ==
  "p{1}" : Inport  PortDimensions=2
  Delays 1 : Subsystem
  "IW{1,1}" : Subsystem
  "b{1}" : Constant  Value=[-7.667554818888461;-7.1506120822451633;6.6095751317742408;-6.0718381124639613;5.486889912285986;-5.0239220460856213;-4.5532354958048833;-3.9686990465867553;-3.3599915866703647;2.9895173488995597;2.4721999146040963;-1.8528559052957085;-1.3285677225896484;-0.8020207022825272;0.26572913489635602;-0.26462999503822782;0.79273760261947346;1.3202657947704826;1.8541270221038295;2.3786283729640085;2.9067837427944707;3.4383648768193251;3.9660324420020445;-4.4901073279672605;5.0159175786220178;-5.5389925625746699;6.0919145231641991;-6.6607382441706715;7.2520973166913469;-7.6649928275821697]
  netsum : Sum  Inputs=2  SaturateOnIntegerOverflow=on  InputSameDT=on  OutDataTypeStr=Inherit: Same as first input
  tansig : neural/Transfer Functions/tansig
  "a{1}" : Outport  InitialOutput=[0;0;0;0;0;0;0;0;0;0;0;0;0;0;0;0;0;0;0;0;0;0;0;0;0;0;0;0;0;0]
  wires:
  "p{1}"/1 -> Delays 1/1("p{1}")
  Delays 1/1("pd{1,1}") -> "IW{1,1}"/1("pd{1,1}")
  "IW{1,1}"/1("iz{1,1}") -> netsum/1
  "b{1}"/1 -> netsum/2
  netsum/1 -> tansig/1
  tansig/1 -> "a{1}"/1

== system hyd_hyb_2_int_cont_Final_AMT/controller1/optimized controller/SOC under 0.5/col_c_d/net_col_c_d_2_4/Layer 2 ==
  "a{1} " : Inport  PortDimensions=30
  Delays 1 : Subsystem
  "LW{2,1}" : Subsystem
  "b{2}" : Constant  Value=[1.5839336690587349;1.50248926749899;-1.3234258824554159;1.363500898088517;-1.2554942744647053;1.1766569011601018;1.0699941283584096;1.0518019010151209;0.93781093147422734;0.86640823154840407;0.80248712442536485;0.73803739217484776;-0.6178465344079328;-0.53340361081275167;-0.43472521333251635;0.36411118131370451;0.22002529446960967;0.17292576820821826;-0.11799416338578383;-0.067696647963401552;0.082233935571546582;-0.097001691420880859;0.20528848140420394;0.30011751510047652;0.37884205091466772;0.41552657082222511;0.52807300796096746;0.62605206644658018;-0.7630299617571652;0.79495876403763588;-0.85134526055578208;0.86915945676567163;-0.98209261069169762;1.1031233054415353;1.1725724745927102;1.2528802540370423;-1.3209599684204105;-1.484229747073051;-1.5264352918712156;1.5588146463980932]
  netsum : Sum  Inputs=2  SaturateOnIntegerOverflow=on  InputSameDT=on  OutDataTypeStr=Inherit: Same as first input
  tansig : neural/Transfer Functions/tansig
  "a{2}" : Outport  InitialOutput=[0;0;0;0;0;0;0;0;0;0;0;0;0;0;0;0;0;0;0;0;0;0;0;0;0;0;0;0;0;0;0;0;0;0;0;0;0;0;0;0]
  wires:
  "a{1} "/1 -> Delays 1/1("p{2}")
  Delays 1/1("pd{2,1}") -> "LW{2,1}"/1("ad{2,1}")
  "LW{2,1}"/1("lz{2,1}") -> netsum/1
  "b{2}"/1 -> netsum/2
  netsum/1 -> tansig/1
  tansig/1 -> "a{2}"/1

== system hyd_hyb_2_int_cont_Final_AMT/controller1/optimized controller/SOC under 0.5/col_c_d/net_col_c_d_2_4/Layer 3 ==
  "a{2} " : Inport  PortDimensions=40
  Delays 1 : Subsystem
  "LW{3,2}" : Subsystem
  "b{3}" : Constant  Value=-0.49177037721686168
  netsum : Sum  Inputs=2  SaturateOnIntegerOverflow=on  InputSameDT=on  OutDataTypeStr=Inherit: Same as first input
  purelin : neural/Transfer Functions/purelin
  "a{3}" : Outport  InitialOutput=0
  wires:
  "a{2} "/1 -> Delays 1/1("p{3}")
  Delays 1/1("pd{3,2}") -> "LW{3,2}"/1("ad{3,2}")
  "LW{3,2}"/1("lz{3,2}") -> netsum/1
  "b{3}"/1 -> netsum/2
  netsum/1 -> purelin/1
  purelin/1 -> "a{3}"/1

== system hyd_hyb_2_int_cont_Final_AMT/controller1/optimized controller/SOC under 0.5/col_c_d/net_col_c_d_2_4/Process Input 1 ==
  x : Inport  PortDimensions=2
  fixunknowns : neural/Processing Functions/fixunknowns  inputSize=2  indices=[1 2]
  mapminmax : neural/Processing Functions/mapminmax  xmin=[0.0059437109537535887;0.46982799999999997]  xmax=[1;0.70796000000000003]  ymin=-1  ymax=1
  removeconstantrows : neural/Processing Functions/removeconstantrows  inputSize=2  keep=[1 2]
  p : Outport  PortDimensions=2
  wires:
  x/1 -> fixunknowns/1
  fixunknowns/1 -> removeconstantrows/1
  removeconstantrows/1 -> mapminmax/1
  mapminmax/1 -> p/1

== system hyd_hyb_2_int_cont_Final_AMT/controller1/optimized controller/SOC under 0.5/col_c_d/net_col_c_d_2_4/Process Output 1 ==
  a : Inport  PortDimensions=1
  mapminmax_reverse : neural/Processing Functions/mapminmax_reverse  xmin=0  xmax=1  ymin=-1  ymax=1
  removeconstantrows_reverse : neural/Processing Functions/removeconstantrows_reverse  inputSize=1  constants=zeros(0,1)  rearrange=1
  y : Outport  PortDimensions=1
  wires:
  a/1 -> mapminmax_reverse/1
  mapminmax_reverse/1 -> removeconstantrows_reverse/1
  removeconstantrows_reverse/1 -> y/1

== system hyd_hyb_2_int_cont_Final_AMT/controller1/optimized controller/SOC under 0.5/col_c_d/net_col_c_d_4_5/Layer 1 ==
  "p{1}" : Inport  PortDimensions=2
  Delays 1 : Subsystem
  "IW{1,1}" : Subsystem
  "b{1}" : Constant  Value=[7.6711565178256951;-7.1288253330240341;6.6225868390307747;-6.0812986301912595;-5.5493083110378478;-5.0213088593936002;-4.5000950323886117;3.9663475145585085;3.4712459058859775;-2.9097981611557908;2.3804784555022125;1.8508616646216531;1.3199022004084437;0.79130835291592105;-0.26571383469130094;0.28169049499133947;0.79750550713874924;-1.3238581719500964;1.8461062666345271;2.3793014464964135;-2.9087862223863818;3.2799361243623686;3.9722610406914955;-4.4951169725581916;5.0242316105510438;5.5527350613983426;6.0841415830313634;-6.608868168673431;7.181227362203801;-7.6405590785617337]
  netsum : Sum  Inputs=2  SaturateOnIntegerOverflow=on  InputSameDT=on  OutDataTypeStr=Inherit: Same as first input
  tansig : neural/Transfer Functions/tansig
  "a{1}" : Outport  InitialOutput=[0;0;0;0;0;0;0;0;0;0;0;0;0;0;0;0;0;0;0;0;0;0;0;0;0;0;0;0;0;0]
  wires:
  "p{1}"/1 -> Delays 1/1("p{1}")
  Delays 1/1("pd{1,1}") -> "IW{1,1}"/1("pd{1,1}")
  "IW{1,1}"/1("iz{1,1}") -> netsum/1
  "b{1}"/1 -> netsum/2
  netsum/1 -> tansig/1
  tansig/1 -> "a{1}"/1

== system hyd_hyb_2_int_cont_Final_AMT/controller1/optimized controller/SOC under 0.5/col_c_d/net_col_c_d_4_5/Layer 2 ==
  "a{1} " : Inport  PortDimensions=30
  Delays 1 : Subsystem
  "LW{2,1}" : Subsystem
  "b{2}" : Constant  Value=[-1.571997776716725;-1.500547923628583;-1.4344144728735191;-1.3485981476129583;1.2532615718144944;-1.1652544395467217;1.155903607831404;1.0204607849765226;0.93992743852922955;-0.85373658974550393;-0.69787475034579782;-0.6824066860868383;0.59227260201826559;-0.52350877795914341;-0.38907007032221552;-0.38354863554124402;0.28867428744586404;-0.17280612608128357;0.081479308809037546;0.042831759023161345;0.027948183126196909;0.11917164457787356;0.17750637593106278;-0.2903026653818756;0.36574660843600959;0.44677726361554676;-0.52228714977647928;-0.61032523248309478;0.67884162446908447;0.74530076353736896;-0.85260059400288024;-0.91415220026869759;-1.0072555741673885;-1.0931119640740525;1.1783975482817304;-1.2572745232766196;1.3404760027268945;1.4151954117700076;-1.497652831876769;1.5845951799704416]
  netsum : Sum  Inputs=2  SaturateOnIntegerOverflow=on  InputSameDT=on  OutDataTypeStr=Inherit: Same as first input
  tansig : neural/Transfer Functions/tansig
  "a{2}" : Outport  InitialOutput=[0;0;0;0;0;0;0;0;0;0;0;0;0;0;0;0;0;0;0;0;0;0;0;0;0;0;0;0;0;0;0;0;0;0;0;0;0;0;0;0]
  wires:
  "a{1} "/1 -> Delays 1/1("p{2}")
  Delays 1/1("pd{2,1}") -> "LW{2,1}"/1("ad{2,1}")
  "LW{2,1}"/1("lz{2,1}") -> netsum/1
  "b{2}"/1 -> netsum/2
  netsum/1 -> tansig/1
  tansig/1 -> "a{2}"/1

== system hyd_hyb_2_int_cont_Final_AMT/controller1/optimized controller/SOC under 0.5/col_c_d/net_col_c_d_4_5/Layer 3 ==
  "a{2} " : Inport  PortDimensions=40
  Delays 1 : Subsystem
  "LW{3,2}" : Subsystem
  "b{3}" : Constant  Value=-0.059572213551021519
  netsum : Sum  Inputs=2  SaturateOnIntegerOverflow=on  InputSameDT=on  OutDataTypeStr=Inherit: Same as first input
  purelin : neural/Transfer Functions/purelin
  "a{3}" : Outport  InitialOutput=0
  wires:
  "a{2} "/1 -> Delays 1/1("p{3}")
  Delays 1/1("pd{3,2}") -> "LW{3,2}"/1("ad{3,2}")
  "LW{3,2}"/1("lz{3,2}") -> netsum/1
  "b{3}"/1 -> netsum/2
  netsum/1 -> purelin/1
  purelin/1 -> "a{3}"/1

== system hyd_hyb_2_int_cont_Final_AMT/controller1/optimized controller/SOC under 0.5/col_c_d/net_col_c_d_4_5/Process Input 1 ==
  x : Inport  PortDimensions=2
  fixunknowns : neural/Processing Functions/fixunknowns  inputSize=2  indices=[1 2]
  mapminmax : neural/Processing Functions/mapminmax  xmin=[0.014616872843449858;0.54464650000000003]  xmax=[1;0.80128200000000005]  ymin=-1  ymax=1
  removeconstantrows : neural/Processing Functions/removeconstantrows  inputSize=2  keep=[1 2]
  p : Outport  PortDimensions=2
  wires:
  x/1 -> fixunknowns/1
  fixunknowns/1 -> removeconstantrows/1
  removeconstantrows/1 -> mapminmax/1
  mapminmax/1 -> p/1

== system hyd_hyb_2_int_cont_Final_AMT/controller1/optimized controller/SOC under 0.5/col_c_d/net_col_c_d_4_5/Process Output 1 ==
  a : Inport  PortDimensions=1
  mapminmax_reverse : neural/Processing Functions/mapminmax_reverse  xmin=0  xmax=1  ymin=-1  ymax=1
  removeconstantrows_reverse : neural/Processing Functions/removeconstantrows_reverse  inputSize=1  constants=zeros(0,1)  rearrange=1
  y : Outport  PortDimensions=1
  wires:
  a/1 -> mapminmax_reverse/1
  mapminmax_reverse/1 -> removeconstantrows_reverse/1
  removeconstantrows_reverse/1 -> y/1

== system hyd_hyb_2_int_cont_Final_AMT/controller1/optimized controller/SOC under 0.5/col_c_d1/net_col_c_d_2_4/Layer 1 ==
  "p{1}" : Inport  PortDimensions=2
  Delays 1 : Subsystem
  "IW{1,1}" : Subsystem
  "b{1}" : Constant  Value=[-7.667554818888461;-7.1506120822451633;6.6095751317742408;-6.0718381124639613;5.486889912285986;-5.0239220460856213;-4.5532354958048833;-3.9686990465867553;-3.3599915866703647;2.9895173488995597;2.4721999146040963;-1.8528559052957085;-1.3285677225896484;-0.8020207022825272;0.26572913489635602;-0.26462999503822782;0.79273760261947346;1.3202657947704826;1.8541270221038295;2.3786283729640085;2.9067837427944707;3.4383648768193251;3.9660324420020445;-4.4901073279672605;5.0159175786220178;-5.5389925625746699;6.0919145231641991;-6.6607382441706715;7.2520973166913469;-7.6649928275821697]
  netsum : Sum  Inputs=2  SaturateOnIntegerOverflow=on  InputSameDT=on  OutDataTypeStr=Inherit: Same as first input
  tansig : neural/Transfer Functions/tansig
  "a{1}" : Outport  InitialOutput=[0;0;0;0;0;0;0;0;0;0;0;0;0;0;0;0;0;0;0;0;0;0;0;0;0;0;0;0;0;0]
  wires:
  tansig/1 -> "a{1}"/1
  netsum/1 -> tansig/1
  "b{1}"/1 -> netsum/2
  "IW{1,1}"/1("iz{1,1}") -> netsum/1
  Delays 1/1("pd{1,1}") -> "IW{1,1}"/1("pd{1,1}")
  "p{1}"/1 -> Delays 1/1("p{1}")

== system hyd_hyb_2_int_cont_Final_AMT/controller1/optimized controller/SOC under 0.5/col_c_d1/net_col_c_d_2_4/Layer 2 ==
  "a{1} " : Inport  PortDimensions=30
  Delays 1 : Subsystem
  "LW{2,1}" : Subsystem
  "b{2}" : Constant  Value=[1.5839336690587349;1.50248926749899;-1.3234258824554159;1.363500898088517;-1.2554942744647053;1.1766569011601018;1.0699941283584096;1.0518019010151209;0.93781093147422734;0.86640823154840407;0.80248712442536485;0.73803739217484776;-0.6178465344079328;-0.53340361081275167;-0.43472521333251635;0.36411118131370451;0.22002529446960967;0.17292576820821826;-0.11799416338578383;-0.067696647963401552;0.082233935571546582;-0.097001691420880859;0.20528848140420394;0.30011751510047652;0.37884205091466772;0.41552657082222511;0.52807300796096746;0.62605206644658018;-0.7630299617571652;0.79495876403763588;-0.85134526055578208;0.86915945676567163;-0.98209261069169762;1.1031233054415353;1.1725724745927102;1.2528802540370423;-1.3209599684204105;-1.484229747073051;-1.5264352918712156;1.5588146463980932]
  netsum : Sum  Inputs=2  SaturateOnIntegerOverflow=on  InputSameDT=on  OutDataTypeStr=Inherit: Same as first input
  tansig : neural/Transfer Functions/tansig
  "a{2}" : Outport  InitialOutput=[0;0;0;0;0;0;0;0;0;0;0;0;0;0;0;0;0;0;0;0;0;0;0;0;0;0;0;0;0;0;0;0;0;0;0;0;0;0;0;0]
  wires:
  tansig/1 -> "a{2}"/1
  netsum/1 -> tansig/1
  "b{2}"/1 -> netsum/2
  "LW{2,1}"/1("lz{2,1}") -> netsum/1
  Delays 1/1("pd{2,1}") -> "LW{2,1}"/1("ad{2,1}")
  "a{1} "/1 -> Delays 1/1("p{2}")

== system hyd_hyb_2_int_cont_Final_AMT/controller1/optimized controller/SOC under 0.5/col_c_d1/net_col_c_d_2_4/Layer 3 ==
  "a{2} " : Inport  PortDimensions=40
  Delays 1 : Subsystem
  "LW{3,2}" : Subsystem
  "b{3}" : Constant  Value=-0.49177037721686168
  netsum : Sum  Inputs=2  SaturateOnIntegerOverflow=on  InputSameDT=on  OutDataTypeStr=Inherit: Same as first input
  purelin : neural/Transfer Functions/purelin
  "a{3}" : Outport  InitialOutput=0
  wires:
  purelin/1 -> "a{3}"/1
  netsum/1 -> purelin/1
  "b{3}"/1 -> netsum/2
  "LW{3,2}"/1("lz{3,2}") -> netsum/1
  Delays 1/1("pd{3,2}") -> "LW{3,2}"/1("ad{3,2}")
  "a{2} "/1 -> Delays 1/1("p{3}")

== system hyd_hyb_2_int_cont_Final_AMT/controller1/optimized controller/SOC under 0.5/col_c_d1/net_col_c_d_2_4/Process Input 1 ==
  x : Inport  PortDimensions=2
  fixunknowns : neural/Processing Functions/fixunknowns  inputSize=2  indices=[1 2]
  mapminmax : neural/Processing Functions/mapminmax  xmin=[0.0059437109537535887;0.46982799999999997]  xmax=[1;0.70796000000000003]  ymin=-1  ymax=1
  removeconstantrows : neural/Processing Functions/removeconstantrows  inputSize=2  keep=[1 2]
  p : Outport  PortDimensions=2
  wires:
  mapminmax/1 -> p/1
  removeconstantrows/1 -> mapminmax/1
  fixunknowns/1 -> removeconstantrows/1
  x/1 -> fixunknowns/1

== system hyd_hyb_2_int_cont_Final_AMT/controller1/optimized controller/SOC under 0.5/col_c_d1/net_col_c_d_2_4/Process Output 1 ==
  a : Inport  PortDimensions=1
  mapminmax_reverse : neural/Processing Functions/mapminmax_reverse  xmin=0  xmax=1  ymin=-1  ymax=1
  removeconstantrows_reverse : neural/Processing Functions/removeconstantrows_reverse  inputSize=1  constants=zeros(0,1)  rearrange=1
  y : Outport  PortDimensions=1
  wires:
  removeconstantrows_reverse/1 -> y/1
  mapminmax_reverse/1 -> removeconstantrows_reverse/1
  a/1 -> mapminmax_reverse/1

== system hyd_hyb_2_int_cont_Final_AMT/controller1/optimized controller/SOC under 0.5/col_c_d1/net_col_c_d_4_5/Layer 1 ==
  "p{1}" : Inport  PortDimensions=2
  Delays 1 : Subsystem
  "IW{1,1}" : Subsystem
  "b{1}" : Constant  Value=[7.6711565178256951;-7.1288253330240341;6.6225868390307747;-6.0812986301912595;-5.5493083110378478;-5.0213088593936002;-4.5000950323886117;3.9663475145585085;3.4712459058859775;-2.9097981611557908;2.3804784555022125;1.8508616646216531;1.3199022004084437;0.79130835291592105;-0.26571383469130094;0.28169049499133947;0.79750550713874924;-1.3238581719500964;1.8461062666345271;2.3793014464964135;-2.9087862223863818;3.2799361243623686;3.9722610406914955;-4.4951169725581916;5.0242316105510438;5.5527350613983426;6.0841415830313634;-6.608868168673431;7.181227362203801;-7.6405590785617337]
  netsum : Sum  Inputs=2  SaturateOnIntegerOverflow=on  InputSameDT=on  OutDataTypeStr=Inherit: Same as first input
  tansig : neural/Transfer Functions/tansig
  "a{1}" : Outport  InitialOutput=[0;0;0;0;0;0;0;0;0;0;0;0;0;0;0;0;0;0;0;0;0;0;0;0;0;0;0;0;0;0]
  wires:
  tansig/1 -> "a{1}"/1
  netsum/1 -> tansig/1
  "b{1}"/1 -> netsum/2
  "IW{1,1}"/1("iz{1,1}") -> netsum/1
  Delays 1/1("pd{1,1}") -> "IW{1,1}"/1("pd{1,1}")
  "p{1}"/1 -> Delays 1/1("p{1}")

== system hyd_hyb_2_int_cont_Final_AMT/controller1/optimized controller/SOC under 0.5/col_c_d1/net_col_c_d_4_5/Layer 2 ==
  "a{1} " : Inport  PortDimensions=30
  Delays 1 : Subsystem
  "LW{2,1}" : Subsystem
  "b{2}" : Constant  Value=[-1.571997776716725;-1.500547923628583;-1.4344144728735191;-1.3485981476129583;1.2532615718144944;-1.1652544395467217;1.155903607831404;1.0204607849765226;0.93992743852922955;-0.85373658974550393;-0.69787475034579782;-0.6824066860868383;0.59227260201826559;-0.52350877795914341;-0.38907007032221552;-0.38354863554124402;0.28867428744586404;-0.17280612608128357;0.081479308809037546;0.042831759023161345;0.027948183126196909;0.11917164457787356;0.17750637593106278;-0.2903026653818756;0.36574660843600959;0.44677726361554676;-0.52228714977647928;-0.61032523248309478;0.67884162446908447;0.74530076353736896;-0.85260059400288024;-0.91415220026869759;-1.0072555741673885;-1.0931119640740525;1.1783975482817304;-1.2572745232766196;1.3404760027268945;1.4151954117700076;-1.497652831876769;1.5845951799704416]
  netsum : Sum  Inputs=2  SaturateOnIntegerOverflow=on  InputSameDT=on  OutDataTypeStr=Inherit: Same as first input
  tansig : neural/Transfer Functions/tansig
  "a{2}" : Outport  InitialOutput=[0;0;0;0;0;0;0;0;0;0;0;0;0;0;0;0;0;0;0;0;0;0;0;0;0;0;0;0;0;0;0;0;0;0;0;0;0;0;0;0]
  wires:
  tansig/1 -> "a{2}"/1
  netsum/1 -> tansig/1
  "b{2}"/1 -> netsum/2
  "LW{2,1}"/1("lz{2,1}") -> netsum/1
  Delays 1/1("pd{2,1}") -> "LW{2,1}"/1("ad{2,1}")
  "a{1} "/1 -> Delays 1/1("p{2}")
